simulink model "WalecOstroslup"  (R2022b)
settings: Solver=VariableStepAuto  StartTime=0.0  StopTime=180  RelTol=1e-3
undefined symbols (not defined in the file): a2, b2, c1, c2, h1i, H2, h20, h2i, kr, L, M, qdiff, qwe, R1, T3
settings Model: Creator=Gabriel  LastModifiedBy=Gabriel
settings SolverCC: InitialStep=10^-6
settings DataIOCC: ReturnWorkspaceOutputs=off

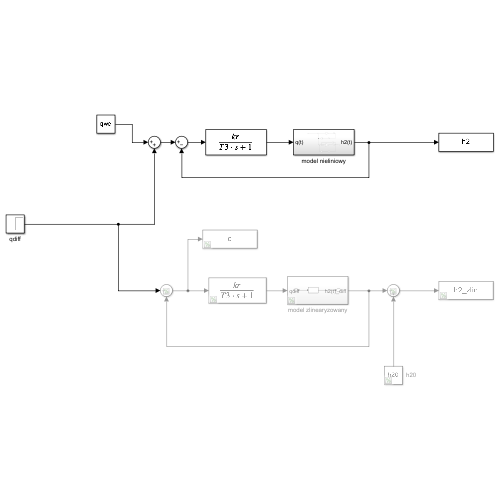
[thumbnail: Simulink's stored preview of the top-level diagram]
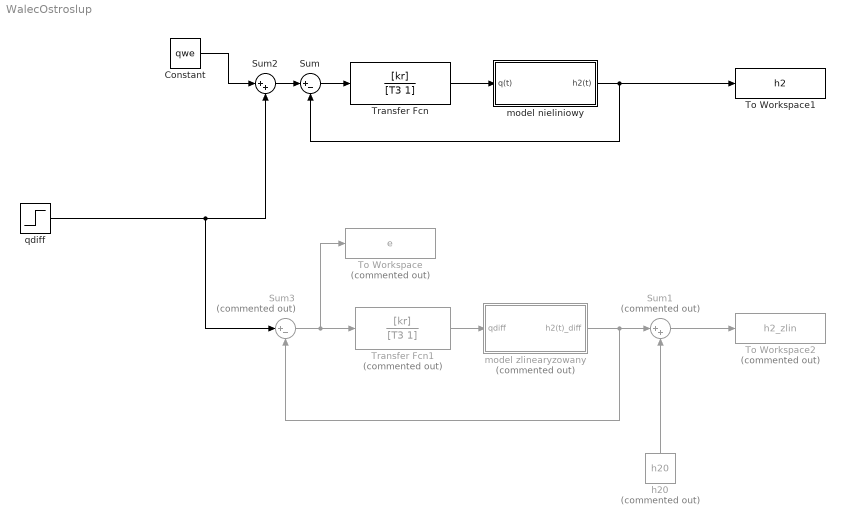
== system WalecOstroslup ==
  Constant : Constant  Value=qwe
  Sum : Sum  Inputs=|+-
  Sum1 : Sum  Commented=on  Inputs=|++
  Sum2 : Sum  Inputs=|++
  Sum3 : Sum  Commented=on  Inputs=|+-
  To Workspace : ToWorkspace  Commented=on  VariableName=e  SaveFormat=Timeseries  SampleTime=10^-3
  To Workspace1 : ToWorkspace  VariableName=h2  SaveFormat=Timeseries  SampleTime=10^-3
  To Workspace2 : ToWorkspace  Commented=on  VariableName=h2_zlin  SaveFormat=Timeseries  SampleTime=10^-3
  Transfer Fcn : TransferFcn  Numerator=[kr]  Denominator=[T3 1]
  Transfer Fcn1 : TransferFcn  Commented=on  Numerator=[kr]  Denominator=[T3 1]
  h20 : Constant  Commented=on  Value=h20
  model nieliniowy : Subsystem
  model zlinearyzowany : Subsystem  Commented=on
  qdiff : Step  Time=0  After=qdiff  SampleTime=0
  wires:
  model zlinearyzowany/1(h2(t)_diff) -> Sum3/2, Sum1/1
  h20/1 -> Sum1/2
  Sum1/1 -> To Workspace2/1
  Transfer Fcn1/1 -> model zlinearyzowany/1(qdiff)
  Sum3/1 -> To Workspace/1, Transfer Fcn1/1
  qdiff/1 -> Sum2/2, Sum3/1
  Constant/1 -> Sum2/1
  model nieliniowy/1(h2(t)) -> To Workspace1/1, Sum/2
  Sum2/1 -> Sum/1
  Sum/1 -> Transfer Fcn/1
  Transfer Fcn/1 -> model nieliniowy/1(q(t))

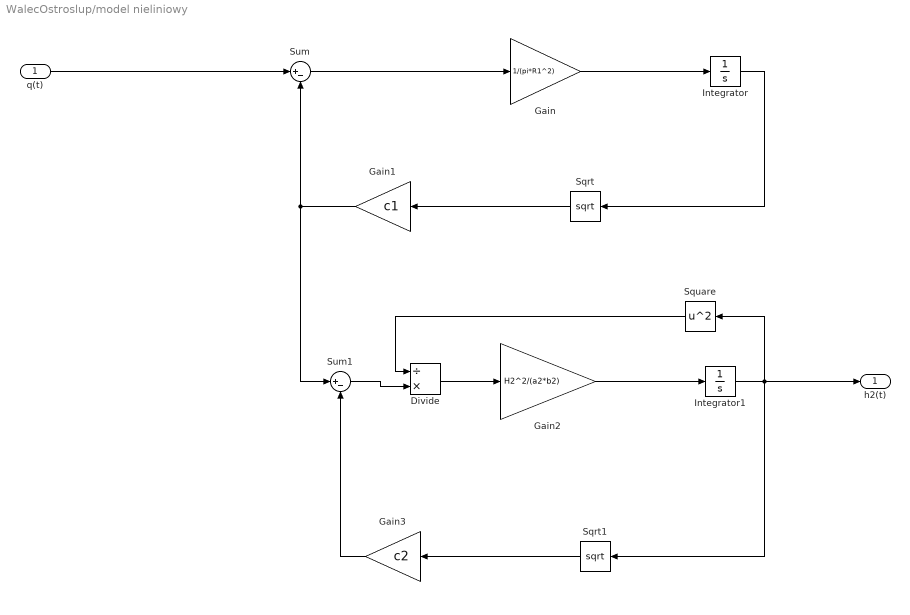
== system WalecOstroslup/model nieliniowy ==
  q(t) : Inport
  Divide : Product  Inputs=/*
  Gain : Gain  Gain=1/(pi*R1^2)
  Gain1 : Gain  Gain=c1
  Gain2 : Gain  Gain=H2^2/(a2*b2)
  Gain3 : Gain  Gain=c2
  Integrator : Integrator  InitialCondition=h1i
  Integrator1 : Integrator  InitialCondition=h2i
  Sqrt : Sqrt
  Sqrt1 : Sqrt
  Square : Math  Operator=square
  Sum : Sum  Inputs=|+-
  Sum1 : Sum  Inputs=|+-
  h2(t) : Outport
  wires:
  Gain1/1 -> Sum/2, Sum1/1
  Sum/1 -> Gain/1
  Sqrt/1 -> Gain1/1
  Integrator1/1 -> h2(t)/1, Square/1, Sqrt1/1
  Square/1 -> Divide/1
  Gain2/1 -> Integrator1/1
  Gain/1 -> Integrator/1
  Divide/1 -> Gain2/1
  Gain3/1 -> Sum1/2
  Sqrt1/1 -> Gain3/1
  Sum1/1 -> Divide/2
  q(t)/1 -> Sum/1
  Integrator/1 -> Sqrt/1

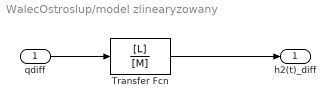
== system WalecOstroslup/model zlinearyzowany ==
  qdiff : Inport
  Transfer Fcn : TransferFcn  Numerator=[L]  Denominator=[M]
  h2(t)_diff : Outport
  wires:
  Transfer Fcn/1 -> h2(t)_diff/1
  qdiff/1 -> Transfer Fcn/1
